simulink model "first_try_model"  (R2020a)
settings: Solver=VariableStepAuto  StartTime=0.0  StopTime=0.05  RelTol=1e-3
libraries: dsparch4 x1
settings Model: Creator=Michael  LastModifiedBy=Michael

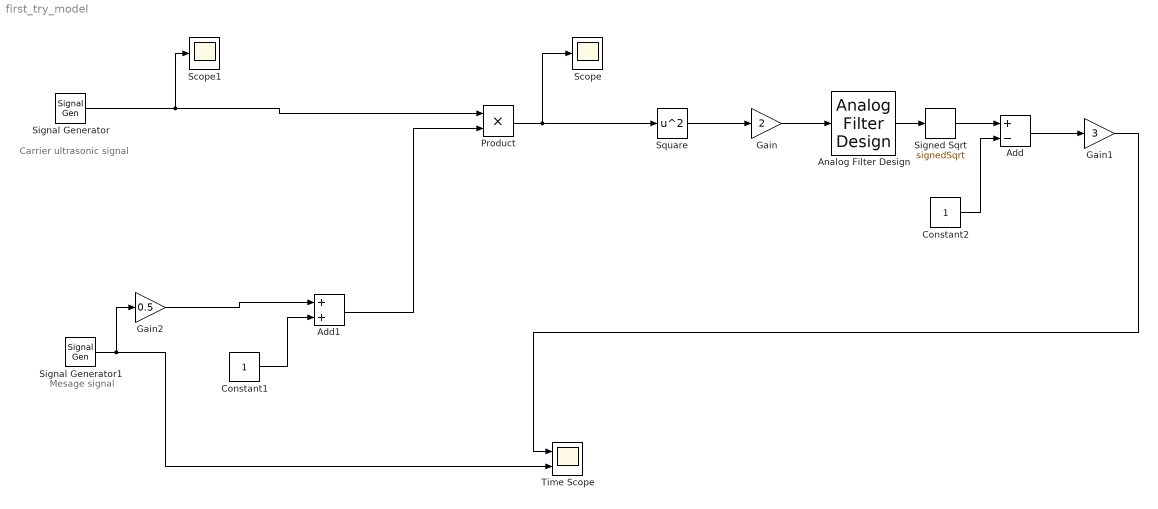
== system first_try_model ==
  note: Mesage signal
  note: Carrier ultrasonic signal
  Add : Sum  Inputs=+-
  Add1 : Sum
  Analog Filter Design : dsparch4/Analog Filter Design  method=Butterworth  filttype=Lowpass  N=10  Wlo=5000  Whi=80  Rp=2  Rs=40
  Constant1 : Constant
  Constant2 : Constant
  Gain : Gain  Gain=2
  Gain1 : Gain  Gain=3
  Gain2 : Gain  Gain=0.5
  Product : Product
  Scope : Scope
  Scope1 : Scope
  Signal Generator : SignalGenerator  Frequency=100000  Units=rad/sec
  Signal Generator1 : SignalGenerator  Frequency=5000  Units=rad/sec
  Signed Sqrt : Sqrt  Operator=signedSqrt  SaturateOnIntegerOverflow=on
  Square : Math  Operator=square  SaturateOnIntegerOverflow=on
  Time Scope : Scope  NumInputPorts=2
  wires:
  Product/1 -> Square/1, Scope/1
  Signal Generator/1 -> Scope1/1, Product/1
  Square/1 -> Gain/1
  Gain/1 -> Analog Filter Design/1
  Constant2/1 -> Add/2
  Add/1 -> Gain1/1
  Gain1/1 -> Time Scope/1
  Signal Generator1/1 -> Gain2/1, Time Scope/2
  Constant1/1 -> Add1/2
  Add1/1 -> Product/2
  Signed Sqrt/1 -> Add/1
  Analog Filter Design/1 -> Signed Sqrt/1
  Gain2/1 -> Add1/1
